simulink model "adaptive_control"  (R2024b)
settings: Solver=VariableStepAuto  StartTime=0.0  StopTime=Tf  FixedStep=0.001  RelTol=1e-3  EnableMultiTasking=on
values from neighbouring files (symbols this model uses):
  a1 = 1    [main.m]
  a2 = 1    [main.m]
  delta_I2hat = 12.12    [main.m]
  delta_m2 = 10    [main.m]
  delta_m2lc2 = 11    [main.m]
  Kd = 750 * eye(n)    [main.m]
  Kpi = 0.01 * eye(8)    [main.m]
  kr1 = 100    [main.m]
  kr2 = 100    [main.m]
  lambda = 5 * eye(n)    [main.m]
  qi = [0; pi/4]    [main.m]
  Tc = 0.005    [main.m]
settings Model: Creator=donato  LastModifiedBy=simy
settings SolverCC: AlgebraicLoopSolver=TrustRegion
settings DataIOCC: ReturnWorkspaceOutputs=off
settings OptimizationCC: LifeSpan=inf
settings DebuggingCC: AlgebraicLoopMsg=none  UnconnectedInputMsg=warning  UnconnectedOutputMsg=warning  UnconnectedLineMsg=warning  SFUnexpectedBacktrackingDiag=warning  SFNoUnconditionalDefaultTransitionDiag=warning  SFExecutionAtInitializationDiag=none  ArithmeticOperatorsInVariantConditions=warning
settings ModelReferenceCC: EnableRefExpFcnMdlSchedulingChecks=on
settings SFSimCC: SimUseLocalCustomCode=off  CustomCodeUndefinedFunction=UseInterfaceOnly
settings RTWCC: RTWUseLocalCustomCode=off  GPUComputeCapability=3.5
settings CodeAppCC: StateflowObjectComments=on
settings GRTTargetCC: TargetLangStandard=C89/C90 (ANSI)
settings ConfigComp: CovMetricSettings=dw  CovSaveCumulativeToWorkspaceVar=on  CovSaveSingleToWorkspaceVar=on  CovExternalEMLEnable=off

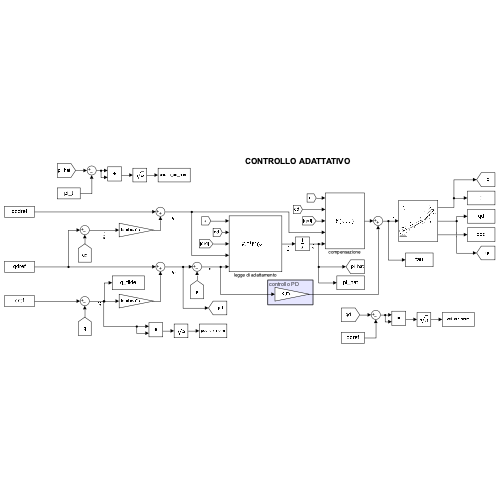
[thumbnail: Simulink's stored preview of the top-level diagram]
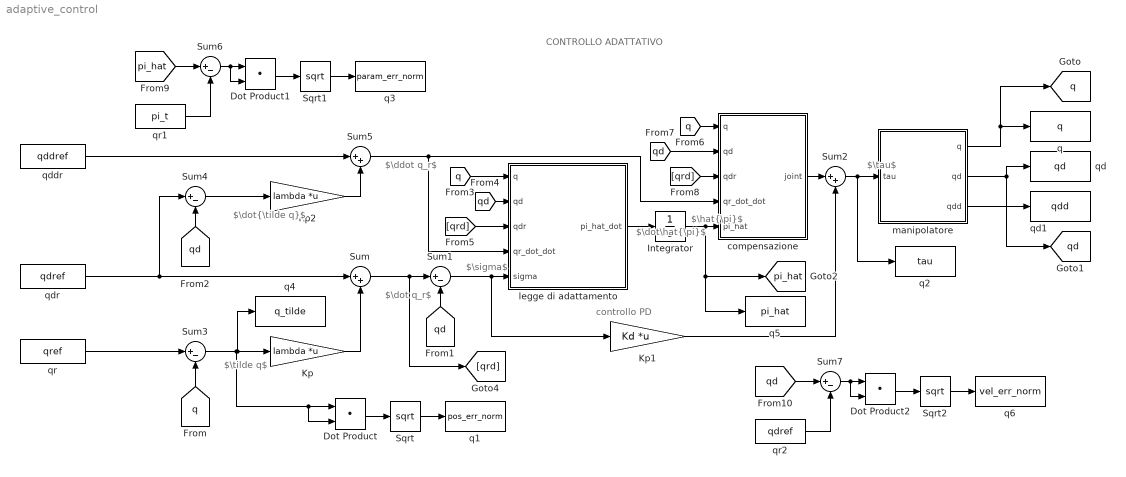
== system adaptive_control ==
  note: controllo PD
  note: $\tilde q$
  note: $\dot q_r$
  note: $\dot\hat{\pi}$
  note: $\sigma$
  note: CONTROLLO ADATTATIVO
  note: $\hat{\pi}$
  note: $\ddot q_r$
  note: $\dot{\tilde q}$
  note: $\tau$
  Dot Product : DotProduct  OutDataTypeStr=Inherit: Inherit via internal rule
  Dot Product1 : DotProduct  OutDataTypeStr=Inherit: Inherit via internal rule
  Dot Product2 : DotProduct  OutDataTypeStr=Inherit: Inherit via internal rule
  Integrator : Integrator  InitialCondition=pi
  Kp : Gain  Gain=lambda  Multiplication=Matrix(K*u)
  Kp1 : Gain  Gain=Kd  Multiplication=Matrix(K*u)
  Kp2 : Gain  Gain=lambda  Multiplication=Matrix(K*u)
  Sqrt : Sqrt
  Sqrt1 : Sqrt
  Sqrt2 : Sqrt
  Sum : Sum  Inputs=|++
  Sum{1,3..4,6..7} (5 alike) : Sum  Inputs=|+-
  Sum2 : Sum  Inputs=|++
  Sum5 : Sum  Inputs=|++
  compensazione : Subsystem
      mask Display: image('Y.png', [0,0,0,0,95,100]);
  legge di adattamento : Subsystem
      mask Display: image('KpiYts.png', [0,0,0,0,99,100]);
  manipolatore : Subsystem
      mask Display: image('manipolatore.png', [0,0,0,0,95,100]);
  q : ToWorkspace  VariableName=q  SampleTime=Tc
  q1 : ToWorkspace  VariableName=pos_err_norm  SampleTime=Tc
  q2 : ToWorkspace  VariableName=tau  SampleTime=Tc
  q3 : ToWorkspace  VariableName=param_err_norm  SampleTime=Tc
  q4 : ToWorkspace  VariableName=q_tilde  SampleTime=Tc
  q5 : ToWorkspace  VariableName=pi_hat  SampleTime=Tc
  q6 : ToWorkspace  VariableName=vel_err_norm  SampleTime=Tc
  qd : ToWorkspace  VariableName=qd  SampleTime=Tc
  qd1 : ToWorkspace  VariableName=qdd  SampleTime=Tc
  qddr : FromWorkspace  VariableName=qddref  SampleTime=Tc
  qdr : FromWorkspace  VariableName=qdref  SampleTime=Tc
  qr : FromWorkspace  VariableName=qref  SampleTime=Tc
  qr1 : FromWorkspace  VariableName=pi_t  SampleTime=Tc
  qr2 : FromWorkspace  VariableName=qdref  SampleTime=Tc
  tag scope: pi_hat=global, q=global, qd=global
  wires:
  manipolatore/1(q) -> q/1, [q]
  manipolatore/2(qd) -> qd/1, [qd]
  manipolatore/3(qdd) -> qd1/1
  qr/1 -> Sum3/1
  qdr/1 -> Sum4/1, Sum/1
  Kp/1 -> Sum/2
  Sum/1 -> Sum1/1, [qrd]
  Sum1/1 -> legge di adattamento/5(sigma), Kp1/1
  Sum2/1 -> manipolatore/1(tau), q2/1
  Kp1/1 -> Sum2/2
  Sum4/1 -> Kp2/1
  qddr/1 -> Sum5/1
  Kp2/1 -> Sum5/2
  Integrator/1 -> q5/1, [pi_hat], compensazione/5(pi_hat)
  [q] -> Sum3/2
  [qd] -> Sum1/2
  [qd] -> Sum4/2
  Sum5/1 -> compensazione/4(qr_dot_dot), legge di adattamento/4(qr_dot_dot)
  [q] -> legge di adattamento/1(q)
  [qd] -> legge di adattamento/2(qd)
  [qrd] -> legge di adattamento/3(qdr)
  legge di adattamento/1(pi_hat_dot) -> Integrator/1
  [q] -> compensazione/1(q)
  [qd] -> compensazione/2(qd)
  [qrd] -> compensazione/3(qdr)
  compensazione/1(joint) -> Sum2/1
  Dot Product/1 -> Sqrt/1
  Sqrt/1 -> q1/1
  Sqrt1/1 -> q3/1
  Dot Product1/1 -> Sqrt1/1
  Sum6/1 -> Dot Product1/2, Dot Product1/1
  [pi_hat] -> Sum6/1
  qr1/1 -> Sum6/2
  Sum3/1 -> Dot Product/2, Dot Product/1, q4/1, Kp/1
  Dot Product2/1 -> Sqrt2/1
  [qd] -> Sum7/1
  qr2/1 -> Sum7/2
  Sqrt2/1 -> q6/1
  Sum7/1 -> Dot Product2/2, Dot Product2/1

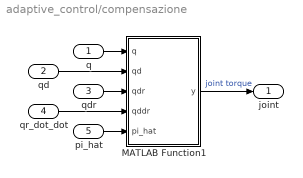
== system adaptive_control/compensazione ==
  q : Inport
  qd : Inport  Port=2
  qdr : Inport  Port=3
  qr_dot_dot : Inport  Port=4
  pi_hat : Inport  Port=5
  MATLAB Function1 : MATLAB Function  TreatAsAtomicUnit=on
  joint : Outport
  wires:
  MATLAB Function1/1(y) -> joint/1  "joint torque"
  qr_dot_dot/1 -> MATLAB Function1/4(qddr)
  qd/1 -> MATLAB Function1/2(qd)
  qdr/1 -> MATLAB Function1/3(qdr)
  pi_hat/1 -> MATLAB Function1/5(pi_hat)
  q/1 -> MATLAB Function1/1(q)

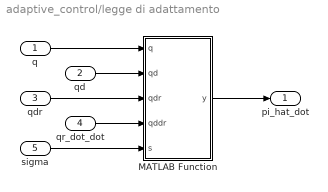
== system adaptive_control/legge di adattamento ==
  q : Inport
  qd : Inport  Port=2
  qdr : Inport  Port=3
  qr_dot_dot : Inport  Port=4
  sigma : Inport  Port=5
  MATLAB Function : MATLAB Function  TreatAsAtomicUnit=on
  pi_hat_dot : Outport
  wires:
  q/1 -> MATLAB Function/1(q)
  qr_dot_dot/1 -> MATLAB Function/4(qddr)
  MATLAB Function/1(y) -> pi_hat_dot/1
  sigma/1 -> MATLAB Function/5(s)
  qdr/1 -> MATLAB Function/3(qdr)
  qd/1 -> MATLAB Function/2(qd)

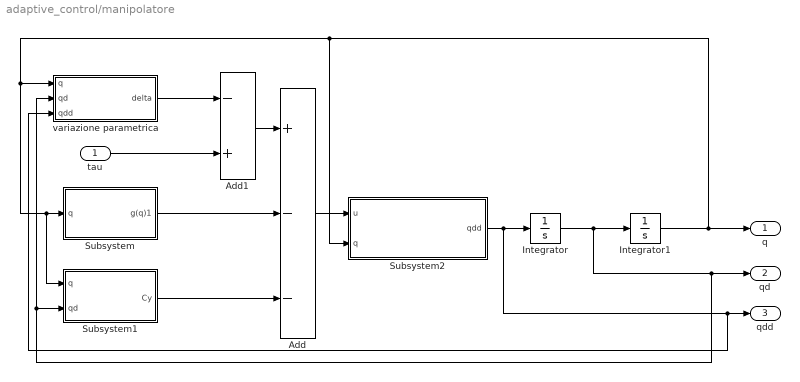
== system adaptive_control/manipolatore ==
  tau : Inport
  Add : Sum  Inputs=+--
  Add1 : Sum  Inputs=-+
  Integrator : Integrator  InitialCondition=[0;0]
  Integrator1 : Integrator  InitialCondition=qi
  Subsystem : Subsystem
      mask Display: image('g.png');
  Subsystem1 : Subsystem
      mask Display: image('C.png');
  Subsystem2 : Subsystem
      mask Display: image('inv_dinamica.png', [0,0,0,0,90,90]);
  variazione parametrica : Subsystem
      mask Display: image('delta.png');
  q : Outport
  qd : Outport  Port=2
  qdd : Outport  Port=3
  wires:
  Integrator/1 -> Integrator1/1, variazione parametrica/2(qd), Subsystem1/2(qd), qd/1
  Integrator1/1 -> q/1, Subsystem2/2(q), variazione parametrica/1(q), Subsystem1/1(q), Subsystem/1(q)
  tau/1 -> Add1/2
  Add1/1 -> Add/1
  Subsystem/1(g(q)1) -> Add/2
  Subsystem1/1(Cy) -> Add/3
  Subsystem2/1(qdd) -> Integrator/1, variazione parametrica/3(qdd), qdd/1
  Add/1 -> Subsystem2/1(u)
  variazione parametrica/1(delta) -> Add1/1

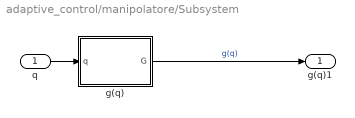
== system adaptive_control/manipolatore/Subsystem ==
  q : Inport
  g(q) : MATLAB Function  TreatAsAtomicUnit=on
  g(q)1 : Outport
  wires:
  g(q)/1(G) -> g(q)1/1  "g(q)"
  q/1 -> g(q)/1(q)

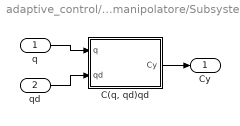
== system adaptive_control/manipolatore/Subsystem1 ==
  q : Inport
  qd : Inport  Port=2
  "C(q, qd)qd" : MATLAB Function  TreatAsAtomicUnit=on
  Cy : Outport
  wires:
  "C(q, qd)qd"/1(Cy) -> Cy/1
  qd/1 -> "C(q, qd)qd"/2(qd)
  q/1 -> "C(q, qd)qd"/1(q)

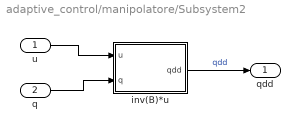
== system adaptive_control/manipolatore/Subsystem2 ==
  u : Inport
  q : Inport  Port=2
  inv(B)*u : MATLAB Function  TreatAsAtomicUnit=on
  qdd : Outport
  wires:
  inv(B)*u/1(qdd) -> qdd/1  "qdd"
  q/1 -> inv(B)*u/2(q)
  u/1 -> inv(B)*u/1(u)

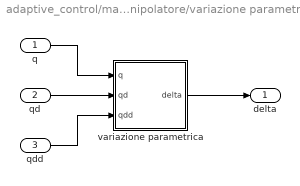
== system adaptive_control/manipolatore/variazione parametrica ==
  q : Inport
  qd : Inport  Port=2
  qdd : Inport  Port=3
  variazione parametrica : MATLAB Function  TreatAsAtomicUnit=on
  delta : Outport
  wires:
  q/1 -> variazione parametrica/1(q)
  qd/1 -> variazione parametrica/2(qd)
  qdd/1 -> variazione parametrica/3(qdd)
  variazione parametrica/1(delta) -> delta/1

== matlab function adaptive_control/compensazione/MATLAB Function1 ==
  data: q input; y output size=[2, 1]; qd input; qdr input; qddr input; pi_hat input; a1 parameter; kr2 parameter; kr1 parameter; a2 parameter
function y = fcn(q, qd, qdr, qddr, pi_hat, a1, kr2, kr1, a2)

    teta1 = q(1); teta2 = q(2); teta1d = qd(1); teta1dr = qdr(1);
    teta2d = qd(2); teta2dr = qdr(2); teta1ddr = qddr(1); teta2ddr = qddr(2);
    c1 = cos(teta1); c2 = cos(teta2); s2 = sin(teta2);
    c12 = cos(teta1 + teta2); g = 9.81;

    y11 = a1^2 * teta1ddr + a1 * g * c1;
    y12 = 2 * a1 * teta1ddr + g * c1;
    y13 = teta1ddr;
    y14 = kr1^2 * teta1ddr;
    y15 = (a1^2 + 2 * a1 * a2 * c2 + a2^2) * teta1ddr + ...
          (a1 * a2 * c2 + a2^2) * teta2ddr - ...
          a1 * a2 * s2 * teta1d * teta2dr - ...
          a1 * a2 * s2 * teta1dr * teta2d - ...
          a1 * a2 * s2 * teta2d * teta2dr + ...
          a1 * g * c1 + a2 * g * c12;
    y16 = (2 * a1 * c2 + 2 * a2) * teta1ddr + ...
          (a1 * c2 + 2 * a2) * teta2ddr - ...
          a1 * s2 * teta1d * teta2dr - ...
          a1 * s2 * teta1dr * teta2d - ...
          a1 * s2 * teta2d * teta2dr + g * c12;
    y17 = teta1ddr + teta2ddr;
    y18 = kr2 * teta2ddr;
    y25 = (a1 * a2 * c2 + a2^2) * teta1ddr + ...
          a2^2 * teta2ddr + a1 * a2 * s2 * teta1d * teta1dr + a2 * g * c12;
    y26 = (a1 * c2 + 2 * a2) * teta1ddr + 2 * a2 * teta2ddr + ...
          a1 * s2 * teta1d * teta1dr + g * c12;
    y27 = teta1ddr + teta2ddr;
    y28 = kr2 * teta1ddr + kr2^2 * teta2ddr;
    Y = [y11 y12 y13 y14 y15 y16 y17 y18;
         0 0 0 0 y25 y26 y27 y28];

    y = Y * pi_hat;
end

== matlab function adaptive_control/legge di adattamento/MATLAB Function ==
  data: q input; qd input; qdr input; qddr input; s input; Kpi parameter; a1 parameter; y output; kr2 parameter; kr1 parameter; a2 parameter
function y  = fcn(q, qd, qdr, qddr, s, Kpi, a1, kr2, kr1, a2)

    teta1 = q(1); teta2 = q(2); teta1d = qd(1); teta1dr = qdr(1);
    teta2d = qd(2); teta2dr = qdr(2); teta1ddr = qddr(1); teta2ddr = qddr(2);
    c1 = cos(teta1); c2 = cos(teta2); s2 = sin(teta2);
    c12 = cos(teta1 + teta2); g = 9.81;

    y11 = a1^2 * teta1ddr + a1 * g * c1;
    y12 = 2 * a1 * teta1ddr + g * c1;
    y13 = teta1ddr;
    y14 = kr1^2 * teta1ddr;
    y15 = (a1^2 + 2 * a1 * a2 * c2 + a2^2) * teta1ddr + ...
          (a1 * a2 * c2 + a2^2) * teta2ddr - ...
          a1 * a2 * s2 * teta1d * teta2dr - ...
          a1 * a2 * s2 * teta1dr * teta2d - ...
          a1 * a2 * s2 * teta2d * teta2dr + ...
          a1 * g * c1 + a2 * g * c12;
    y16 = (2 * a1 * c2 + 2 * a2) * teta1ddr + ...
          (a1 * c2 + 2 * a2) * teta2ddr - ...
          a1 * s2 * teta1d * teta2dr - ...
          a1 * s2 * teta1dr * teta2d - ...
          a1 * s2 * teta2d * teta2dr + g * c12;
    y17 = teta1ddr + teta2ddr;
    y18 = kr2 * teta2ddr;
    y25 = (a1 * a2 * c2 + a2^2) * teta1ddr + ...
          a2^2 * teta2ddr + a1 * a2 * s2 * teta1d * teta1dr + a2 * g * c12;
    y26 = (a1 * c2 + 2 * a2) * teta1ddr + 2 * a2 * teta2ddr + ...
          a1 * s2 * teta1d * teta1dr + g * c12;
    y27 = teta1ddr + teta2ddr;
    y28 = kr2 * teta1ddr + kr2^2 * teta2ddr;
    Y = [y11 y12 y13 y14 y15 y16 y17 y18;
         0 0 0 0 y25 y26 y27 y28];

    y = Kpi \ (Y' * s);
end

== matlab function adaptive_control/manipolatore/Subsystem/g(q) ==
  data: q input; G output size=[2, 1]
function G = fcn(q)
    
    a1 = 1; l1 = 0.5; l2 = 0.5; ml1 = 50; ml2 = 50; mm2 = 5; g = 9.81; 
    teta1 = q(1); teta2 = q(2); c1 = cos(teta1); c12 = cos(teta1 + teta2);

    g1 = (ml1 * l1 + mm2 * a1 + ml2 * a1) * g * c1 + ml2 * l2 * g * c12;
    g2 = ml2 * l2 * g * c12;
    G = [g1;
         g2];
end

== matlab function adaptive_control/manipolatore/Subsystem1/C(q, qd)qd ==
  data: q input; Cy output size=[2, 1]; qd input
function Cy = fcn(q, qd)
    a1 = 1; l2 = 0.5; ml2 = 50; 
    teta2 = q(2); teta1d = qd(1); teta2d = qd(2); s2 = sin(teta2); 

    h = -ml2 * a1 * l2 * s2;
    C = [h*teta2d h*(teta1d+teta2d); -h*teta1d 0];
    Cy = C * qd;
end

== matlab function adaptive_control/manipolatore/Subsystem2/inv(B)*u ==
  data: u input; qdd output size=[2, 1]; q input
function qdd = fcn(u, q)
    a1 = 1; l1 = 0.5; l2 = 0.5; ml1 = 50; ml2 = 50; Il1 = 10; Il2 = 10; 
    kr1 = 100; kr2 = 100; mm2 = 5; Im1 = 0.01; Im2 = 0.01;

    teta2 = q(2); c2 = cos(teta2); 

    b11 = Il1 + ml1 * l1^2 + kr1^2 * Im1 + Il2 + ...
          ml2 * (a1^2 + l2^2 + 2 * a1 * l2 *c2) + Im2 + mm2 * a1^2;
    b12 = Il2 + ml2 * (l2^2 + a1 * l2 * c2) + kr2 * Im2;
    b21 = b12;
    b22 = Il2 + ml2 * l2^2 + kr2^2 * Im2;
    B = [b11 b12; b21 b22];

    qdd = B \ u;
end

== matlab function adaptive_control/manipolatore/variazione parametrica/variazione parametrica ==
  data: q input; delta output; qd input; qdd input; a1 parameter; a2 parameter; delta_m2 parameter; delta_m2lc2 parameter; delta_I2hat parameter
function delta = fcn(q, qd, qdd, a1, a2, delta_m2, delta_m2lc2, delta_I2hat)
    teta1 = q(1); teta2 = q(2); teta1d = qd(1); 
    teta2d = qd(2); teta1dd = qdd(1); teta2dd = qdd(2);
    c1 = cos(teta1); c2 = cos(teta2); s2 = sin(teta2);
    c12 = cos(teta1 + teta2); g = 9.81;

    y15 = (a1^2 + 2 * a1 * a2 * c2 + a2^2) * teta1dd + ...
          (a1 * a2 * c2 + a2^2) * teta2dd - ...
          2 * a1 * a2 * s2 * teta1d * teta2d - ...
          a1 * a2 * s2 * teta2d^2 + ...
          a1 * g * c1 + a2 * g * c12;
    y16 = (2 * a1 * c2 + 2 * a2) * teta1dd + ...
          (a1 * c2 + 2 * a2) * teta2dd - ...
          2 * a1 * s2 * teta1d * teta2d - ...
          a1 * s2 * teta2d^2 + g * c12;
    y17 = teta1dd + teta2dd;
    y25 = (a1 * a2 * c2 + a2^2) * teta1dd + ...
          a2^2 * teta2dd + a1 * a2 * s2 * teta1d^2 + a2 * g * c12;
    y26 = (a1 * c2 + 2 * a2) * teta1dd + 2 * a2 * teta2dd + ...
          a1 * s2 * teta1d^2 + g * c12;
    y27 = teta1dd + teta2dd;
    Y = [0 0 0 0 y15 y16 y17 0;
         0 0 0 0 y25 y26 y27 0];

    pi = [0 0 0 0 delta_m2 delta_m2lc2 delta_I2hat 0]';

    delta = Y * pi;
end
